simulink model "controlSystem_PowerScope"  (R2021a)
settings: Solver=VariableStepAuto  StartTime=0.0  StopTime=50  RelTol=1e-7
undefined symbols (not defined in the file): initialFuel, maxEngineTemp, maxEngineTorque, maxMotorTemp, maxMotorTorque, maxRegenTorque, motorVoltage, sigbuilder_block
libraries: autolibshared x6, autolibsharedcoupling x3, autolibhevctrlrcommon x2, autolibutils x2, autolibmappedmotor x2, autolibshareddiff x1, autolibtransamt x1, autolibdcdc x1, autolibdatasheetbattery x1, autolibsharedmappedengines x1
(part 1 of 5)
settings Model: EnablePacing=on  PacingRate=10  Creator=peter  LastModifiedBy=nwdep
settings DebuggingCC: SFMachineParentedDataDiag=warning

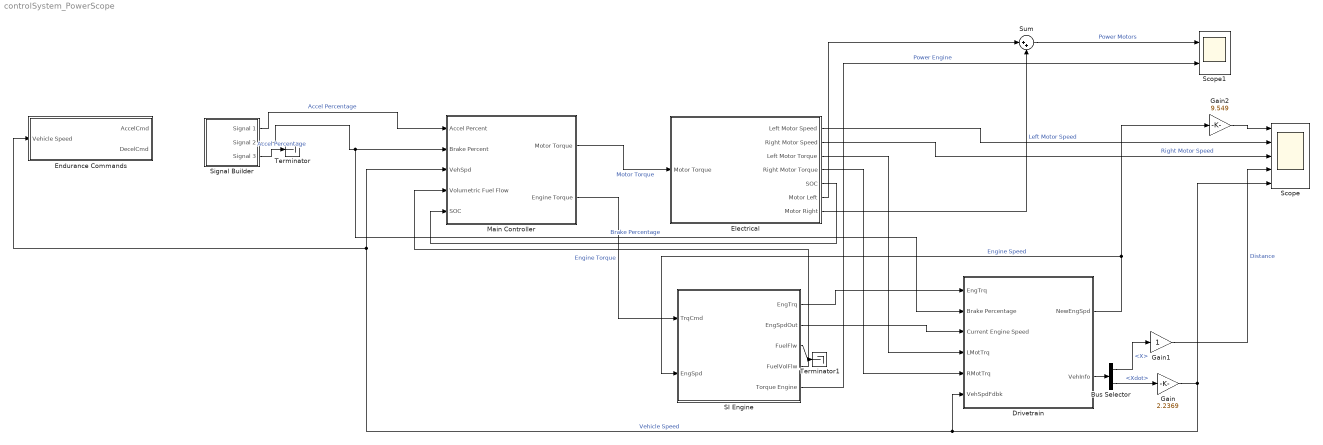
== system controlSystem_PowerScope ==
  Bus Selector : BusSelector  OutputSignals=InertFrm.Cg.Disp.X,InertFrm.Cg.Vel.Xdot
  Drivetrain : Subsystem
  Electrical : Subsystem
  Endurance Commands : Subsystem
  Gain : Gain  Gain=2.2369
  Gain1 : Gain
  Gain2 : Gain  Gain=9.549
  Main Controller : Subsystem
  SI Engine : Subsystem
  Scope : Scope  NumInputPorts=5
  Scope1 : Scope  NumInputPorts=2
  Signal Builder : Subsystem  Tag=STV Subsys  LoadFcn=sigbuilder_block('load');  StartFcn=sigbuilder_block('start');  StopFcn=sigbuilder_block('stop');  ClipboardFcn=sigbuilder_block('clipboard');  mask(Sigbuilder block){tuvar=[0:10]}
      mask help: Simulink:masks:SigbuilderBlock_MD
      mask init:
      | if ~strcmp(get_param(bdroot(gcbh),'SimulationStatus'),'stopped') tuvar = sigbuilder_block('maskInit'); end
      settings: CopyFcn=sigbuilder_block('copy');  DeleteFcn=sigbuilder_block('delete');  ModelCloseFcn=sigbuilder_block('modelClose');  PreSaveFcn=sigbuilder_block('preSave');  PauseFcn=sigbuilder_block('pause');  ContinueFcn=sigbuilder_block('continue');  NameChangeFcn=sigbuilder_block('namechange');  OpenFcn=sigbuilder_block('open',[334.2 75 550.8 400.2 ]);  CloseFcn=sigbuilder_block('close');
      mask Display: plot(0, 0, 100, 100,[2, 2, 32, 32, 2], [68, 8, 8, 68, 68],[32, 2], [38, 38], [32, 19, 2],[53, 60, 44], [32, 17, 17, 2],[16, 16, 31, 31]);txt = getActiveGroup(gcbh);text(2, 100, txt,'verticalAlignment', 'top');
  Sum : Sum  Inputs=|++
  Terminator : Terminator
  Terminator1 : Terminator
  wires:
  Electrical/5(SOC) -> Main Controller/5(SOC)
  Main Controller/1(Motor Torque) -> Electrical/1(Motor Torque)  "Motor Torque"
  Main Controller/2(Engine Torque) -> SI Engine/1(TrqCmd)  "Engine Torque"
  Drivetrain/1(NewEngSpd) -> Gain2/1, SI Engine/2(EngSpd)  "Engine Speed"
  SI Engine/3(FuelFlw) -> Terminator1/1
  SI Engine/4(FuelVolFlw) -> Main Controller/4(Volumetric Fuel Flow)
  SI Engine/2(EngSpdOut) -> Drivetrain/3(Current Engine Speed)
  SI Engine/1(EngTrq) -> Drivetrain/1(EngTrq)
  Electrical/3(Left Motor Torque) -> Drivetrain/4(LMotTrq)
  Electrical/4(Right Motor Torque) -> Drivetrain/5(RMotTrq)
  Electrical/1(Left Motor Speed) -> Scope/2  "Left Motor Speed"
  Electrical/2(Right Motor Speed) -> Scope/3  "Right Motor Speed"
  Drivetrain/2(VehInfo) -> Bus Selector/1
  Bus Selector/1 -> Gain1/1  "<X>"
  Bus Selector/2 -> Gain/1  "<Xdot>"
  Gain/1 -> Scope/5, Endurance Commands/1(Vehicle Speed), Main Controller/3(VehSpd), Drivetrain/6(VehSpdFdbk)  "Vehicle Speed"
  Gain1/1 -> Scope/4  "Distance"
  Gain2/1 -> Scope/1
  Signal Builder/3(Signal 3) -> Terminator/1  "Accel Percentage"
  Signal Builder/2(Signal 2) -> Drivetrain/2(Brake Percentage), Main Controller/2(Brake Percent)  "Brake Percentage"
  Signal Builder/1(Signal 1) -> Main Controller/1(Accel Percent)  "Accel Percentage"
  SI Engine/5(Torque Engine) -> Scope1/2  "Power Engine"
  Electrical/6(Motor Left) -> Sum/1
  Electrical/7(Motor Right) -> Sum/2
  Sum/1 -> Scope1/1  "Power Motors"

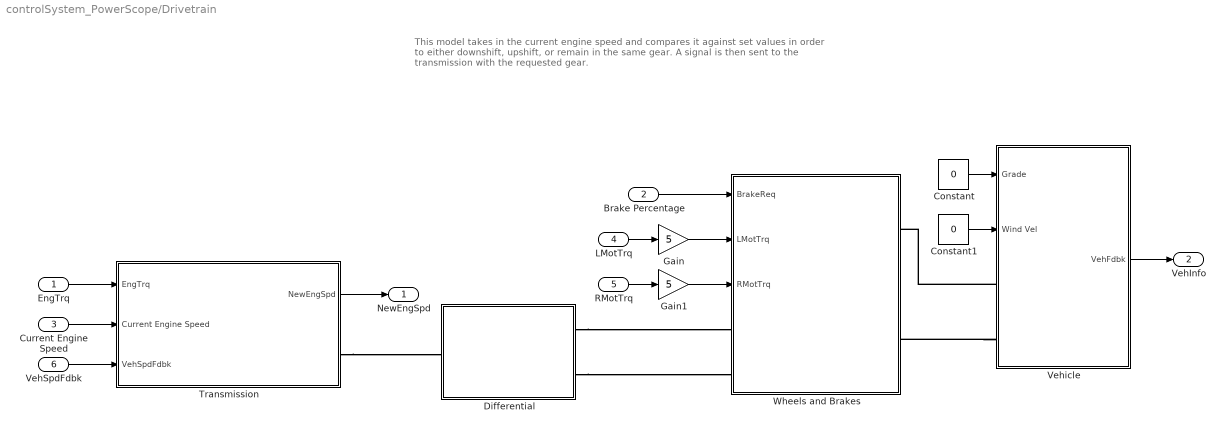
== system controlSystem_PowerScope/Drivetrain ==
  note: This model takes in the current engine speed and compares it against set values in order to either downshift, upshift, or remain in the same gear. A signal is then sent to the transmission with the requested gear.
  EngTrq : Inport
  Brake Percentage : Inport  Port=2
  Current Engine Speed : Inport  Port=3
  LMotTrq : Inport  Port=4
  RMotTrq : Inport  Port=5
  VehSpdFdbk : Inport  Port=6
  Constant : Constant  Value=0
  Constant1 : Constant  Value=0
  Differential : Subsystem
  Gain : Gain  Gain=5
  Gain1 : Gain  Gain=5
  Transmission : Subsystem
  Vehicle : Subsystem
  Wheels and Brakes : Subsystem  VariantControl=0
  NewEngSpd : Outport
  VehInfo : Outport  Port=2
  wires:
  Constant/1 -> Vehicle/1(Grade)
  Constant1/1 -> Vehicle/2(Wind Vel)
  Brake Percentage/1 -> Wheels and Brakes/1(BrakeReq)
  EngTrq/1 -> Transmission/1(EngTrq)
  Current Engine Speed/1 -> Transmission/2(Current Engine Speed)
  VehSpdFdbk/1 -> Transmission/3(VehSpdFdbk)
  Transmission/1(NewEngSpd) -> NewEngSpd/1
  Vehicle/1(VehFdbk) -> VehInfo/1
  LMotTrq/1 -> Gain/1
  RMotTrq/1 -> Gain1/1
  Gain/1 -> Wheels and Brakes/2(LMotTrq)
  Gain1/1 -> Wheels and Brakes/3(RMotTrq)
  connections:
  Vehicle/LConn2 -- Wheels and Brakes/RConn2
  Transmission/RConn1 -- Differential/LConn1
  Differential/RConn1 -- Wheels and Brakes/LConn1
  Differential/RConn2 -- Wheels and Brakes/LConn2
  Vehicle/LConn1 -- Wheels and Brakes/RConn1

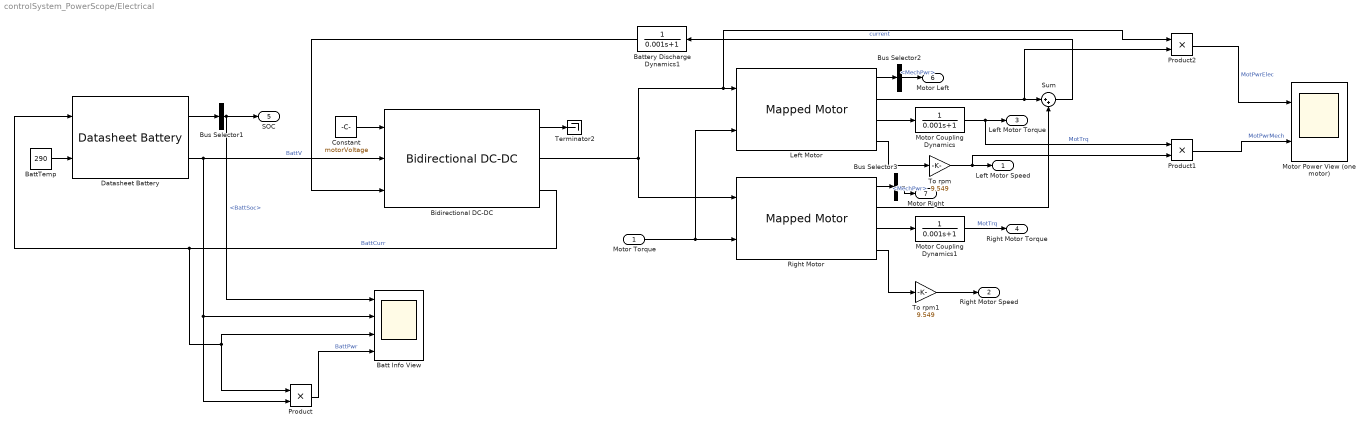
== system controlSystem_PowerScope/Electrical ==
  Motor Torque : Inport
  " Right Motor" : autolibmappedmotor/Mapped Motor  port_config=Torque  param_by=Tabulated torque-speed envelope  w_t=motorSpeeds  T_t=motorTorques  torque_max=80  power_max=30000  Tc=0.02  param_loss=Tabulated efficiency data  eff=88  w_eff=419  T_eff=26  Piron=0  Pbase=0  w_eff_bp=motorSpeeds  T_eff_bp=[0 8 16 24 32 40 48 56 64 72 80]  Temp_eff_bp=[233.15 293.15 373.15]  losses_table=[1.49 1.67 2.21 3.10; 0.42 0.69 1.14 2.03; 0.06 0.24 0.78 1.68; 0.42 0.69 1.14 2.03; 1.49 1.67 2.21 3.10]  losses_table_3d=cat(3,1.05*[1.49 1.67 2.21 3.10; 0.42 0.69 1.14 2.03; 0.06 0.24 0.78 1.68; 0.42 0.69 1.14 2.03; 1.49 1.67 2.21 3.10],[1.49 1.67 2.21 3.10; 0.42 0.69 1.14 2.03; 0.06 0.24 0.78 1.68; 0.42 0.69 1.14 2.03; 1.49 1.67 2.21 3.10],1.03*[1.49 1.67 2.21 3.10; 0.42 0.69 1.14 2.03; 0.06 0.24 0.78 1.68; 0.42 0.69 1.14 2.03; 1.49 1.67 2.21 3.10])  efficiency_table=|  efficiency_table_3d=cat(3,90*ones(5,4),95*ones(5,4),92*ones(5,4))  J=.042  b=.042  omega_o=0  T_t_extended=[40.93 44.07 47.75 52.09 57.3 63.66 71.62 80 80 80 80 80 80 80 80 80 80 80 80 80 80 80 71.62 63.66 57.3 52.09 47.75 44.07 40.93]  w_t_extended=[-733.038285837618 -680.678408277789 -628.318530717959 -575.958653158129 -523.598775598299 -471.238898038469 -418.879020478639 -374.999123017327 -314.159265358979 -261.799387799149 -209.43951023932 -157.07963267949 -104.71975511966 -52.3598775598299 0 52.3598775598299 104.71975511966 157.07963267949 209.43951023932 261.799387799149 314.159265358979 374.999123017327 418.879020478639 471.238898038469 523.598775598299 575.958653158129 628.318530717959 680.678408277789 733.038285837618]  KLossIron=0  KLossCopper=2.1976  x_w_eff_vec=[-733.038285837618 -680.678408277789 -628.318530717959 -575.958653158129 -523.598775598299 -471.238898038469 -418.879020478639 -374.999123017327 -314.159265358979 -261.799387799149 -209.43951023932 -157.07963267949 -104.71975511966 -52.3598775598299 0 52.3598775598299 104.71975511966 157.07963267949 209.43951023932 261.799387799149 314.159265358979 374.999123017327 418.879020478639 471.238898038469 523.598775598299 575.958653158129 628.318530717959 680.678408277789 733.038285837618]  x_T_eff_vec=[-80 -72 -64 -56 -48 -40 -32 -24 -16 -8 0 8 16 24 32 40 48 56 64 72 80]  x_tmp_eff_vec=[233.15 293.15 373.15]  x_losses_mat=[4413.99397923727 3972.59458131354 3531.19518338981 3089.79578546609 2648.39638754236 2206.99698961863 1765.59759169491 1324.19819377118 1159.97267209469 954.654511788527 0 821.002880138133 1055.57513160617 1231.5043202072 1642.00576027626 2052.50720034533 2463.0086404144 2873.51008048346 3284.01152055253 3694.51296062159 4105.01440069066;4098.70869500603 3688.83782550543 3278.96695600483 2869.09608650422 2459.22521700362 2049.35434750302 1639.48347800241 1229.61260850181 1077.11748123078 886.464903803632 0 762.359817271123 980.176907920015 1143.53972590668 1524.71963454225 1905.89954317781 2287.07945181337 2668.25936044893 3049.43926908449 3430.61917772005 3811.79908635561;3783.4234107748 3405.08106969732 3026.73872861984 2648.39638754236 2270.05404646488 1891.7117053874 1513.36936430992 1135.02702323244 874.182303607594 818.275295818737 0 703.716754404114 804.247719318987 1055.57513160617 1407.43350880823 1759.29188601028 2111.15026321234 2463.0086404144 2814.86701761645 3166.72539481851 3518.58377202057;3468.13812654357 3121.32431388921 2774.51050123485 2427.6966885805 2080.88287592614 1734.06906327178 1387.25525061743 1040.44143796307 801.333778306961 750.085687833842 0 645.073691537104 737.227076042404 967.610537305655 1290.14738307421 1612.68422884276 1935.22107461131 2257.75792037986 2580.29476614841 2902.83161191697 3225.36845768552;3152.85284231233 2837.5675580811 2522.28227384987 2206.99698961863 1891.7117053874 1576.42642115617 1261.14113692493 945.8558526937 828.551908639065 681.896079848948 0 586.430628670095 753.98223686155 879.645943005141 1172.86125734019 1466.07657167524 1759.29188601028 2052.50720034533 2345.72251468038 2638.93782901542 2932.15314335047;2837.5675580811 2553.81080227299 2270.05404646488 1986.29729065677 1702.54053484866 1418.78377904055 1135.02702323244 851.27026742433 745.696717775159 613.706471864053 0 527.787565803085 678.584013175395 791.681348704627 1055.57513160617 1319.46891450771 1583.36269740925 1847.2564803108 2111.15026321234 2375.04404611388 2638.93782901542;2522.28227384987 2270.05404646488 2017.82581907989 1765.59759169491 1513.36936430992 1261.14113692493 1165.57640481013 874.182303607594 744.673814184248 638.291840729355 0 536.165146212658 670.206432765822 804.247719318987 1072.33029242532 1172.86125734019 1407.43350880823 1642.00576027626 1876.5780117443 2111.15026321234 2345.72251468038;2258.05923537315 2032.25331183583 1806.44738829852 1580.6414647612 1354.83554122389 1304.34477571244 1186.81041130758 890.107808480687 818.179904765078 658.53504529872 0 539.998737144951 719.998316193268 809.998105717426 1079.9974742899 1199.99719365545 1259.99705333822 1469.99656222792 1679.99607111762 1889.99558000733 2099.99508889703;2485.6557259172 2237.09015332548 1748.36460721519 1529.81903131329 1311.27345541139 1242.8278629586 994.262290366878 837.758040957278 685.438397146865 551.694319654793 0 452.38934211693 603.18578948924 753.98223686155 904.77868423386 1130.97335529233 1206.37157897848 1407.43350880823 1608.49543863797 2035.75203952619 2261.94671058465;2855.99332144527 2570.39398930074 2284.79465715621 1628.97396852804 1396.26340159546 1163.55283466289 930.842267730309 856.797996433581 681.896079848948 523.598775598299 0 418.879020478639 586.430628670095 753.98223686155 837.758040957278 1047.1975511966 1256.63706143592 1466.07657167524 2010.61929829747 2261.94671058465 2513.27412287183;2727.58431939579 2454.82588745621 2182.06745551663 1599.35626000935 1370.87679429373 1142.39732857811 913.917862862486 685.438397146864 545.516863879158 418.879020478639 0 335.103216382911 469.144502936076 603.18578948924 804.247719318987 1005.30964914873 1206.37157897848 1407.43350880823 1876.5780117443 2111.15026321234 2345.72251468038;2393.59440273508 2154.23496246157 1636.55059163747 1431.98176768279 1028.1575957203 856.797996433581 685.438397146865 613.706471864053 409.137647909369 314.159265358979 0 251.327412287183 351.858377202057 527.787565803085 603.18578948924 753.98223686155 ...(+5556 chars)]  x_losses_mat_3d=cat(3,[3.255 2.3205 1.7535 1.5645 1.7535 2.3205 3.255;2.1315 1.197 0.7245 0.441 0.7245 1.197 2.1315;1.764 0.819 0.252 0.063 0.252 0.819 1.764;2.1315 1.197 0.7245 0.441 0.7245 1.197 2.1315;3.255 2.3205 1.7535 1.5645 1.7535 2.3205 3.255],[3.1 2.21 1.67 1.49 1.67 2.21 3.1;2.03 1.14 0.69 0.42 0.69 1.14 2.03;1.68 0.78 0.24 0.06 0.24 0.78 1.68;2.03 1.14 0.69 0.42 0.69 1.14 2.03;3.1 2.21 1.67 1.49 1.67 2.21 3.1],[3.193 2.2763 1.7201 1.5347 1.7201 2.2763 3.193;2.0909 1.1742 0.7107 0.4326 0.7107 1.1742 2.0909;1.7304 0.8034 0.2472 0.0618 0.2472 0.8034 1.7304;2.0909 1.1742 0.7107 0.4326 0.7107 1.1742 2.0909;3.193 2.2763 1.7201 1.5347 1.7201 2.2763 3.193])  CalLossMapData={}  CalLossWithTempMapData={}  aMode=2  RefBlkName='autolibmappedmotor/Mapped Motor'
      | [52 78 80 82 82 80 78 78 76 74 70; 52 78 80 82 82 80 78 78 76 74 70; 52 78 84 86 86 86 86 84 84 82 82; 52 80 86 86 88 88 88 86 86 84 84; 52 80 86 88 88 88 88 88 86 86 86;
      | 52 80 86 88 90 90 90 90 88 88 88; 52 82 88 90 91 91 92 92 92 91 91;
      | 52 82 88 91 91 92 93 93 93 93 93;
      | 52 84 90 92 92 93 93 93 93 93 93; 62 86 91 93 93 93 93 93 93 93 93;
      | 66 86 91 93 93 93 93 93 93 93 93; 70 86 92 93 93 93 93 93 93 93 93; 70 86 92 93 93 93 93 93 93 93 93;
      | 72 86 91 93 93 93 93 93 93 93 93;
      | 72 86 91 93 93 93 93 93 93 93 93]
      settings: SourceProductBaseCode=PW,DR,MT,UV,VE
  Batt Info View : Scope  NumInputPorts=4
  BattTemp : Constant  Value=290
  Battery Discharge Dynamics1 : TransferFcn  Denominator=[0.001 1]
  Bidirectional DC-DC : autolibdcdc/Bidirectional DC-DC  Tc=1/1000  Vinit=motorVoltage  Plimit=30000  param_loss=Single efficiency measurement  eff=98  v_loss_bp=[0 200 400 600 800 1000]  i_loss_bp=[0 25 50 75 100]  losses_table=[100 100 100 100 100;100 150 200 250 300;100 200 300 400 500;100 250 400 550 700;100 300 500 700 900;100 350 600 850 1100]  v_eff_bp=[200 400 600 800 1000]  i_eff_bp=[25 50 75 100]  efficiency_table=[96.2 98.1 98.7 99;98.1 99 99.4 99.5;98.7 99.4 99.6 99.7;99 99.5 99.7 99.8;99.2 99.6 99.7 99.8]  x_v_bp=[-1000 -800 -600 -400 -200 200 400 600 800 1000]  x_i_bp=[-100 -75 -50 -25 25 50 75 100]  x_losses_mat=[200.400801603196 225.67703109328 200.803212851408 201.612903225806 199.999999999997 200 225 200;160.320641282556 180.541624874624 201.005025125625 202.020202020203 200 200 180 160;180.541624874624 180.722891566267 181.086519114686 197.568389057748 194.999999999999 179.999999999997 180 180;201.005025125625 181.086519114686 202.020202020203 193.67991845056 190 200 179.999999999997 200;202.020202020203 197.568389057748 193.67991845056 197.505197505197 190 190 194.999999999999 200;200 194.999999999999 190 190 197.505197505197 193.67991845056 197.568389057748 202.020202020203;200 179.999999999997 200 190 193.67991845056 202.020202020203 181.086519114686 201.005025125625;180 180 179.999999999997 194.999999999999 197.568389057748 181.086519114686 180.722891566267 180.541624874624;160 180 200 200 202.020202020203 201.005025125625 180.541624874624 160.320641282556;200 225 200 199.999999999997 201.612903225806 200.803212851408 225.67703109328 200.400801603196]  RefBlkName='autolibdcdc/Bidirectional DC-DC'
      settings: SourceProductBaseCode=PW
  Bus Selector1 : BusSelector  OutputSignals=BattSoc
  Bus Selector2 : BusSelector  OutputSignals=MechPwr
  Bus Selector3 : BusSelector  OutputSignals=MechPwr
  Constant : Constant  Value=motorVoltage
  Datasheet Battery : autolibdatasheetbattery/Datasheet Battery  CapacityCtrl=Parameter  OutputVlt=Filtered  BattChargeMax=2.5  Em=[2.8 3.228 3.284 3.361 3.408 3.427 3.472 3.477 3.493 3.504 3.516 3.528 3.537 3.545 3.555 3.561 3.566 3.576 3.587 3.589 3.594 3.6 3.608 3.61 3.616 3.619 3.626 3.632 3.637 3.64 3.645 3.646 3.652 3.655 3.658 3.661 3.664 3.668 3.673 3.678 3.68 3.681 3.686 3.692 3.699 3.702 3.705 3.71 3.717 3.723 3.728 3.733 3.735 3.742 3.749 3.755 3.761 3.768 3.773 3.78 3.791 3.798 3.798 3.814 3.818 3.825 3.841 3.846 3.855 3.863 3.877 3.885 3.894 3.907 3.919 3.926 3.935 3.944 3.954 3.964 3.974 3.988 3.998 4.014 4.029 4.034 4.047 4.065 4.074 4.086 4.097 4.131 4.126 4.138 4.15 4.18 4.174 4.187 4.207 4.231 4.221]  CapLUTBp=[0 0.01 0.02 0.03 0.04 0.05 0.06 0.07 0.08 0.09 0.1 0.11 0.12 0.13 0.14 0.15 0.16 0.17 0.18 0.19 0.2 0.21 0.22 0.23 0.24 0.25 0.26 0.27 0.28 0.29 0.3 0.31 0.32 0.33 0.34 0.35 0.36 0.37 0.38 0.39 0.4 0.41 0.42 0.43 0.44 0.45 0.46 0.47 0.48 0.49 0.5 0.51 0.52 0.53 0.54 0.55 0.56 0.57 0.58 0.59 0.6 0.61 0.62 0.63 0.64 0.65 0.66 0.67 0.68 0.69 0.7 0.71 0.72 0.73 0.74 0.75 0.76 0.77 0.78 0.79 0.8 0.81 0.82 0.83 0.84 0.85 0.86 0.87 0.88 0.89 0.9 0.91 0.92 0.93 0.94 0.95 0.96 0.97 0.98 0.99 1]  RInt=[0.008846 0.009319 0.009027 0.00847 0.01032 0.01314;0.006389 0.006554 0.005553 0.005525 0.006043 0.007805;0.004364 0.004101 0.00406 0.003452 0.003846 0.004517;0.002031 0.002563 0.002532 0.00246 0.002716 0.003047;0.001443 0.001825 0.001795 0.001778 0.001924 0.002234;0.0005603 0.0007192 0.0006887 0.0007557 0.0007355 0.001014;0.001028 0.001338 0.001 0.001536 0.001546 0.002789]  BattTempBp=[243.1 253.1 263.1 273.1 283.1 298.1 313.1]  CapSOCBp=[0 0.2 0.4 0.6 0.8 1]  Ns=32  Np=9  BattCapInit=2.5  Tc=1/1000  Vinit=4.221  RefBlkName='autolibdatasheetbattery/Datasheet Battery'
      settings: SourceProductBaseCode=PW
  Left Motor : autolibmappedmotor/Mapped Motor  port_config=Torque  param_by=Tabulated torque-speed envelope  w_t=motorSpeeds  T_t=motorTorques  torque_max=80  power_max=30000  Tc=0.02  param_loss=Tabulated efficiency data  eff=88  w_eff=419  T_eff=26  Piron=0  Pbase=0  w_eff_bp=motorSpeeds  T_eff_bp=[0 8 16 24 32 40 48 56 64 72 80]  Temp_eff_bp=[233.15 293.15 373.15]  losses_table=[1.49 1.67 2.21 3.10; 0.42 0.69 1.14 2.03; 0.06 0.24 0.78 1.68; 0.42 0.69 1.14 2.03; 1.49 1.67 2.21 3.10]  losses_table_3d=cat(3,1.05*[1.49 1.67 2.21 3.10; 0.42 0.69 1.14 2.03; 0.06 0.24 0.78 1.68; 0.42 0.69 1.14 2.03; 1.49 1.67 2.21 3.10],[1.49 1.67 2.21 3.10; 0.42 0.69 1.14 2.03; 0.06 0.24 0.78 1.68; 0.42 0.69 1.14 2.03; 1.49 1.67 2.21 3.10],1.03*[1.49 1.67 2.21 3.10; 0.42 0.69 1.14 2.03; 0.06 0.24 0.78 1.68; 0.42 0.69 1.14 2.03; 1.49 1.67 2.21 3.10])  efficiency_table=|  efficiency_table_3d=cat(3,90*ones(5,4),95*ones(5,4),92*ones(5,4))  J=.042  b=.042  omega_o=0  T_t_extended=[40.93 44.07 47.75 52.09 57.3 63.66 71.62 80 80 80 80 80 80 80 80 80 80 80 80 80 80 80 71.62 63.66 57.3 52.09 47.75 44.07 40.93]  w_t_extended=[-733.038285837618 -680.678408277789 -628.318530717959 -575.958653158129 -523.598775598299 -471.238898038469 -418.879020478639 -374.999123017327 -314.159265358979 -261.799387799149 -209.43951023932 -157.07963267949 -104.71975511966 -52.3598775598299 0 52.3598775598299 104.71975511966 157.07963267949 209.43951023932 261.799387799149 314.159265358979 374.999123017327 418.879020478639 471.238898038469 523.598775598299 575.958653158129 628.318530717959 680.678408277789 733.038285837618]  KLossIron=0  KLossCopper=2.1976  x_w_eff_vec=[-733.038285837618 -680.678408277789 -628.318530717959 -575.958653158129 -523.598775598299 -471.238898038469 -418.879020478639 -374.999123017327 -314.159265358979 -261.799387799149 -209.43951023932 -157.07963267949 -104.71975511966 -52.3598775598299 0 52.3598775598299 104.71975511966 157.07963267949 209.43951023932 261.799387799149 314.159265358979 374.999123017327 418.879020478639 471.238898038469 523.598775598299 575.958653158129 628.318530717959 680.678408277789 733.038285837618]  x_T_eff_vec=[-80 -72 -64 -56 -48 -40 -32 -24 -16 -8 0 8 16 24 32 40 48 56 64 72 80]  x_tmp_eff_vec=[233.15 293.15 373.15]  x_losses_mat=[4413.99397923727 3972.59458131354 3531.19518338981 3089.79578546609 2648.39638754236 2206.99698961863 1765.59759169491 1324.19819377118 1159.97267209469 954.654511788527 0 821.002880138133 1055.57513160617 1231.5043202072 1642.00576027626 2052.50720034533 2463.0086404144 2873.51008048346 3284.01152055253 3694.51296062159 4105.01440069066;4098.70869500603 3688.83782550543 3278.96695600483 2869.09608650422 2459.22521700362 2049.35434750302 1639.48347800241 1229.61260850181 1077.11748123078 886.464903803632 0 762.359817271123 980.176907920015 1143.53972590668 1524.71963454225 1905.89954317781 2287.07945181337 2668.25936044893 3049.43926908449 3430.61917772005 3811.79908635561;3783.4234107748 3405.08106969732 3026.73872861984 2648.39638754236 2270.05404646488 1891.7117053874 1513.36936430992 1135.02702323244 874.182303607594 818.275295818737 0 703.716754404114 804.247719318987 1055.57513160617 1407.43350880823 1759.29188601028 2111.15026321234 2463.0086404144 2814.86701761645 3166.72539481851 3518.58377202057;3468.13812654357 3121.32431388921 2774.51050123485 2427.6966885805 2080.88287592614 1734.06906327178 1387.25525061743 1040.44143796307 801.333778306961 750.085687833842 0 645.073691537104 737.227076042404 967.610537305655 1290.14738307421 1612.68422884276 1935.22107461131 2257.75792037986 2580.29476614841 2902.83161191697 3225.36845768552;3152.85284231233 2837.5675580811 2522.28227384987 2206.99698961863 1891.7117053874 1576.42642115617 1261.14113692493 945.8558526937 828.551908639065 681.896079848948 0 586.430628670095 753.98223686155 879.645943005141 1172.86125734019 1466.07657167524 1759.29188601028 2052.50720034533 2345.72251468038 2638.93782901542 2932.15314335047;2837.5675580811 2553.81080227299 2270.05404646488 1986.29729065677 1702.54053484866 1418.78377904055 1135.02702323244 851.27026742433 745.696717775159 613.706471864053 0 527.787565803085 678.584013175395 791.681348704627 1055.57513160617 1319.46891450771 1583.36269740925 1847.2564803108 2111.15026321234 2375.04404611388 2638.93782901542;2522.28227384987 2270.05404646488 2017.82581907989 1765.59759169491 1513.36936430992 1261.14113692493 1165.57640481013 874.182303607594 744.673814184248 638.291840729355 0 536.165146212658 670.206432765822 804.247719318987 1072.33029242532 1172.86125734019 1407.43350880823 1642.00576027626 1876.5780117443 2111.15026321234 2345.72251468038;2258.05923537315 2032.25331183583 1806.44738829852 1580.6414647612 1354.83554122389 1304.34477571244 1186.81041130758 890.107808480687 818.179904765078 658.53504529872 0 539.998737144951 719.998316193268 809.998105717426 1079.9974742899 1199.99719365545 1259.99705333822 1469.99656222792 1679.99607111762 1889.99558000733 2099.99508889703;2485.6557259172 2237.09015332548 1748.36460721519 1529.81903131329 1311.27345541139 1242.8278629586 994.262290366878 837.758040957278 685.438397146865 551.694319654793 0 452.38934211693 603.18578948924 753.98223686155 904.77868423386 1130.97335529233 1206.37157897848 1407.43350880823 1608.49543863797 2035.75203952619 2261.94671058465;2855.99332144527 2570.39398930074 2284.79465715621 1628.97396852804 1396.26340159546 1163.55283466289 930.842267730309 856.797996433581 681.896079848948 523.598775598299 0 418.879020478639 586.430628670095 753.98223686155 837.758040957278 1047.1975511966 1256.63706143592 1466.07657167524 2010.61929829747 2261.94671058465 2513.27412287183;2727.58431939579 2454.82588745621 2182.06745551663 1599.35626000935 1370.87679429373 1142.39732857811 913.917862862486 685.438397146864 545.516863879158 418.879020478639 0 335.103216382911 469.144502936076 603.18578948924 804.247719318987 1005.30964914873 1206.37157897848 1407.43350880823 1876.5780117443 2111.15026321234 2345.72251468038;2393.59440273508 2154.23496246157 1636.55059163747 1431.98176768279 1028.1575957203 856.797996433581 685.438397146865 613.706471864053 409.137647909369 314.159265358979 0 251.327412287183 351.858377202057 527.787565803085 603.18578948924 753.98223686155 ...(+5556 chars)]  x_losses_mat_3d=cat(3,[3.255 2.3205 1.7535 1.5645 1.7535 2.3205 3.255;2.1315 1.197 0.7245 0.441 0.7245 1.197 2.1315;1.764 0.819 0.252 0.063 0.252 0.819 1.764;2.1315 1.197 0.7245 0.441 0.7245 1.197 2.1315;3.255 2.3205 1.7535 1.5645 1.7535 2.3205 3.255],[3.1 2.21 1.67 1.49 1.67 2.21 3.1;2.03 1.14 0.69 0.42 0.69 1.14 2.03;1.68 0.78 0.24 0.06 0.24 0.78 1.68;2.03 1.14 0.69 0.42 0.69 1.14 2.03;3.1 2.21 1.67 1.49 1.67 2.21 3.1],[3.193 2.2763 1.7201 1.5347 1.7201 2.2763 3.193;2.0909 1.1742 0.7107 0.4326 0.7107 1.1742 2.0909;1.7304 0.8034 0.2472 0.0618 0.2472 0.8034 1.7304;2.0909 1.1742 0.7107 0.4326 0.7107 1.1742 2.0909;3.193 2.2763 1.7201 1.5347 1.7201 2.2763 3.193])  CalLossMapData={}  CalLossWithTempMapData={}  aMode=2  RefBlkName='autolibmappedmotor/Mapped Motor'
      | [52 78 80 82 82 80 78 78 76 74 70; 52 78 80 82 82 80 78 78 76 74 70; 52 78 84 86 86 86 86 84 84 82 82; 52 80 86 86 88 88 88 86 86 84 84; 52 80 86 88 88 88 88 88 86 86 86;
      | 52 80 86 88 90 90 90 90 88 88 88; 52 82 88 90 91 91 92 92 92 91 91;
      | 52 82 88 91 91 92 93 93 93 93 93;
      | 52 84 90 92 92 93 93 93 93 93 93; 62 86 91 93 93 93 93 93 93 93 93;
      | 66 86 91 93 93 93 93 93 93 93 93; 70 86 92 93 93 93 93 93 93 93 93; 70 86 92 93 93 93 93 93 93 93 93;
      | 72 86 91 93 93 93 93 93 93 93 93;
      | 72 86 91 93 93 93 93 93 93 93 93]
      settings: SourceProductBaseCode=PW,DR,MT,UV,VE
  Motor Coupling Dynamics : TransferFcn  Denominator=[0.001 1]
  Motor Coupling Dynamics1 : TransferFcn  Denominator=[0.001 1]
  Motor Power View (one motor) : Scope  NumInputPorts=2
  Product : Product
  Product1 : Product
  Product2 : Product
  Sum : Sum  Inputs=|++
  Terminator2 : Terminator
  To rpm : Gain  Gain=9.549
  To rpm1 : Gain  Gain=9.549
  Left Motor Speed : Outport
  Right Motor Speed : Outport  Port=2
  Left Motor Torque : Outport  Port=3
  Right Motor Torque : Outport  Port=4
  SOC : Outport  Port=5
  Motor Left : Outport  Port=6
  Motor Right : Outport  Port=7
  wires:
  BattTemp/1 -> Datasheet Battery/2
  Datasheet Battery/1 -> Bus Selector1/1
  Left Motor/2 -> Product2/2, Sum/1
  " Right Motor"/4 -> To rpm1/1
  " Right Motor"/2 -> Sum/2
  Bus Selector1/1 -> Batt Info View/1, SOC/1  "<BattSoc>"
  " Right Motor"/1 -> Bus Selector3/1
  Left Motor/1 -> Bus Selector2/1
  Motor Torque/1 -> Left Motor/2, " Right Motor"/2
  Sum/1 -> Battery Discharge Dynamics1/1  "current"
  Left Motor/3 -> Motor Coupling Dynamics/1
  Motor Coupling Dynamics/1 -> Product1/1, Left Motor Torque/1  "MotTrq"
  " Right Motor"/3 -> Motor Coupling Dynamics1/1
  Motor Coupling Dynamics1/1 -> Right Motor Torque/1  "MotTrq"
  Bidirectional DC-DC/2 -> Product2/1, Left Motor/1, " Right Motor"/1
  Datasheet Battery/2 -> Bidirectional DC-DC/2, Product/2, Batt Info View/2  "BattV"
  Constant/1 -> Bidirectional DC-DC/1
  Bidirectional DC-DC/3 -> Product/1, Batt Info View/3, Datasheet Battery/1  "BattCurr"
  Battery Discharge Dynamics1/1 -> Bidirectional DC-DC/3
  Bidirectional DC-DC/1 -> Terminator2/1
  To rpm1/1 -> Right Motor Speed/1
  Left Motor/4 -> To rpm/1
  To rpm/1 -> Product1/2, Left Motor Speed/1
  Product/1 -> Batt Info View/4  "BattPwr"
  Product1/1 -> Motor Power View (one motor)/2  "MotPwrMech"
  Product2/1 -> Motor Power View (one motor)/1  "MotPwrElec"
  Bus Selector2/1 -> Motor Left/1  "<MechPwr>"
  Bus Selector3/1 -> Motor Right/1  "<MechPwr>"

== system controlSystem_PowerScope/Endurance Commands ==
  Vehicle Speed : Inport
  Constant : Constant  Value=0
  Drive Cycle Source : autolibshared/Drive Cycle Source  cycleVar=FTP75  fileVar=cycleFTP75.mat  tfinal="2474  seconds"  cycleRepeat=off  outAccPort=off  outGearPort=off  gearList=No gear data  t_wot1=5  xdot_woto=0  xdot_wot1=30  t_wot2=20  xdot_wot2=0  t_wotend=30  srcUnit=m/s  outUnit=m/s  srcAccUnit=m/s/s  outAccUnit=m/s^2  dt=0  aMode=2  faultOption=off  velBnd=2  velBndUnit=mph  inUnit=m/s  timeBnd=1  failOption=off  stopSim=off  maxFaultCnt=10  maxFaultTime=2  maxTotFaultTime=15  traceOption=off  dtTrace=1  traceWindow=10  lastDCname=FTP75  lastOutUnit=mph  lastDT=0  lastTB=1  lastSB=2  forceCalcBound=off
      settings: SourceProductBaseCode=PW,DR,MT,UV,VE
  Longitudinal Driver : autolibshared/Longitudinal Driver  extAccelOvr=off  extDecelOvr=off  extAccelHld=off  extDecelHld=off  extAccelZero=off  extDecelZero=off  cntrlType=PI  shftType=None  velUnits=m/s  gearOut=off  Kp=10  Ki=5  Kff=.1  Kg=0  VehVelVec=[0 100]  KffVec=[.1 .1]  KpVec=[10 10]  KiVec=[5 5]  KgVec=[0 0]  m=1500  Kpt=3000  tau=.1  L=2  aR=200  bR=2.5  cR=.5  g=9.81  vnom=5  Kaw=1  tauerr=.01  tauPt=2  GearInit=0  tShift=.1  pdlVec=[0.1 0.4 0.5 0.9]  upShftTbl=[-1 12.9375 26.4375 39.9375 51.18749999999999 62.4375 72.84375 83.25;-1 16.3125 29.8125 43.3125 54.5624 65.8125 76.78125 87.75;-1 19.6875 33.1875 46.68749999999999 57.9375 69.1875 80.71875 92.25;-1 33 52.5 77.25 100.5 138.75 161.875 185]  dwnShftTbl=[1 9.5625 23.0625 36.5625 47.8125 59.0625 68.90625 78.75;1 12.9375 26.4375 39.9375 51.18749999999999 62.4375 72.84375 83.25;1 16.3125 29.8125 43.3125 54.562499 65.8125 76.78125 87.75;1 19.6875 33.1875 46.68749999999999 57.9375 69.1875 80.71875 92.25]  tClutch=.5  tRev=.5  tPark=120  aMode=2  UpGearVec="[0  1  2  3  4  5  6  7]"  DownGearVec="[1  2  3  4  5  6  7  8]"
      settings: SourceProductBaseCode=PW,DR,MT,UV,VE
  Terminator4 : Terminator
  AccelCmd : Outport
  DecelCmd : Outport  Port=2
  wires:
  Vehicle Speed/1 -> Longitudinal Driver/2
  Constant/1 -> Longitudinal Driver/3
  Drive Cycle Source/1 -> Longitudinal Driver/1
  Longitudinal Driver/2 -> AccelCmd/1
  Longitudinal Driver/1 -> Terminator4/1
  Longitudinal Driver/3 -> DecelCmd/1

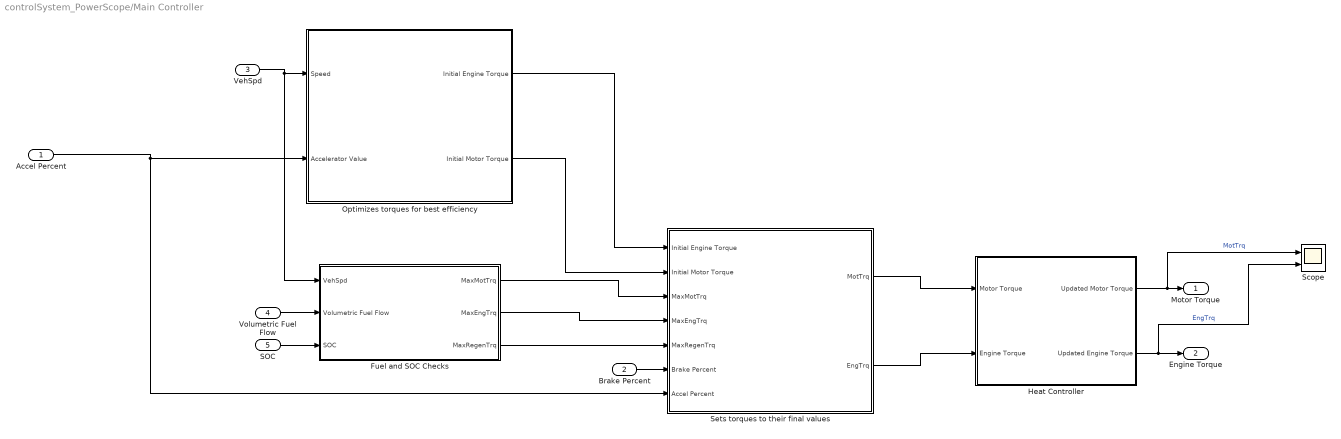
== system controlSystem_PowerScope/Main Controller ==
  Accel Percent : Inport
  Brake Percent : Inport  Port=2
  VehSpd : Inport  Port=3
  Volumetric Fuel Flow : Inport  Port=4
  SOC : Inport  Port=5
  Fuel and SOC Checks : Subsystem
  Heat Controller : Subsystem
  Optimizes torques for best efficiency : Subsystem
  Scope : Scope  NumInputPorts=2
  Sets torques to their final values : Subsystem
  Motor Torque : Outport
  Engine Torque : Outport  Port=2
  wires:
  Accel Percent/1 -> Sets torques to their final values/7(Accel Percent), Optimizes torques for best efficiency/2(Accelerator Value)
  VehSpd/1 -> Optimizes torques for best efficiency/1(Speed), Fuel and SOC Checks/1(VehSpd)
  Volumetric Fuel Flow/1 -> Fuel and SOC Checks/2(Volumetric Fuel Flow)
  SOC/1 -> Fuel and SOC Checks/3(SOC)
  Heat Controller/1(Updated Motor Torque) -> Scope/1, Motor Torque/1  "MotTrq"
  Heat Controller/2(Updated Engine Torque) -> Scope/2, Engine Torque/1  "EngTrq"
  Optimizes torques for best efficiency/1(Initial Engine Torque) -> Sets torques to their final values/1(Initial Engine Torque)
  Optimizes torques for best efficiency/2(Initial Motor Torque) -> Sets torques to their final values/2(Initial Motor Torque)
  Fuel and SOC Checks/1(MaxMotTrq) -> Sets torques to their final values/3(MaxMotTrq)
  Fuel and SOC Checks/2(MaxEngTrq) -> Sets torques to their final values/4(MaxEngTrq)
  Fuel and SOC Checks/3(MaxRegenTrq) -> Sets torques to their final values/5(MaxRegenTrq)
  Brake Percent/1 -> Sets torques to their final values/6(Brake Percent)
  Sets torques to their final values/1(MotTrq) -> Heat Controller/1(Motor Torque)
  Sets torques to their final values/2(EngTrq) -> Heat Controller/2(Engine Torque)
